simulink library "BF_MASTER"  (Simulink 8.6)
settings: Solver=ode45  StartTime=0.0  StopTime=10.0  RelTol=1e-3
libraries: cdsEpicsOut x60, cdsFilt x51, cdsFiltCtrl x28, cdsTP x28, cdsEpicsIn x14, cdsMuxMatrix x6, VIS_LIB x5, cdsEpicsBinIn x3, cdsOsc x2, cdsFunctionCall x2, SIXOSEM_F_STAGE_MASTER x2, CRYP_IM_MASTER x1
(part 5 of 9)

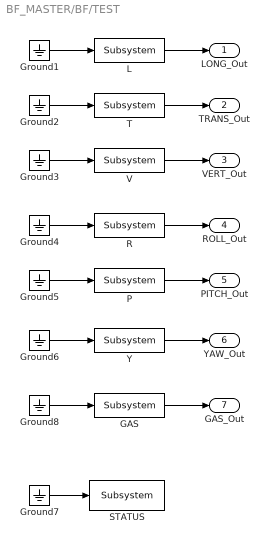
== system BF_MASTER/BF/TEST ==
  GAS : cdsFilt/Subsystem  Tag=cdsFilt  Description=|
      | Purpose:                                                                                                                                                                                                                                  
      | Standard CDS IIR filter module.                                                                                                                                                                                                           
      |                                                                                                                                                                                                                                           
      | Operation:                                                                                                                                                                                                                                
      | Consists of 10 second order section IIR filters, plus a ramped gain stage. In FE code, also provides pre-defined test points and excitation channel inputs. The filter coefficients are defined in the LIGO system using the 'foton' tool.
      |                                                                                                                                                                                                                                           
      | Usage:                                                                                                                                                                                                                                    
      | Name the part with the desired filter module name.
      settings: AttributesFormatString=%<Tag>
  Ground{1..8} (8 alike) : Ground
  L : cdsFilt/Subsystem  Tag=cdsFilt  Description=|
      | Purpose:                                                                                                                                                                                                                                  
      | Standard CDS IIR filter module.                                                                                                                                                                                                           
      |                                                                                                                                                                                                                                           
      | Operation:                                                                                                                                                                                                                                
      | Consists of 10 second order section IIR filters, plus a ramped gain stage. In FE code, also provides pre-defined test points and excitation channel inputs. The filter coefficients are defined in the LIGO system using the 'foton' tool.
      |                                                                                                                                                                                                                                           
      | Usage:                                                                                                                                                                                                                                    
      | Name the part with the desired filter module name.
      settings: AttributesFormatString=%<Tag>
  P : cdsFilt/Subsystem  Tag=cdsFilt  Description=|
      | Purpose:                                                                                                                                                                                                                                  
      | Standard CDS IIR filter module.                                                                                                                                                                                                           
      |                                                                                                                                                                                                                                           
      | Operation:                                                                                                                                                                                                                                
      | Consists of 10 second order section IIR filters, plus a ramped gain stage. In FE code, also provides pre-defined test points and excitation channel inputs. The filter coefficients are defined in the LIGO system using the 'foton' tool.
      |                                                                                                                                                                                                                                           
      | Usage:                                                                                                                                                                                                                                    
      | Name the part with the desired filter module name.
      settings: AttributesFormatString=%<Tag>
  R : cdsFilt/Subsystem  Tag=cdsFilt  Description=|
      | Purpose:                                                                                                                                                                                                                                  
      | Standard CDS IIR filter module.                                                                                                                                                                                                           
      |                                                                                                                                                                                                                                           
      | Operation:                                                                                                                                                                                                                                
      | Consists of 10 second order section IIR filters, plus a ramped gain stage. In FE code, also provides pre-defined test points and excitation channel inputs. The filter coefficients are defined in the LIGO system using the 'foton' tool.
      |                                                                                                                                                                                                                                           
      | Usage:                                                                                                                                                                                                                                    
      | Name the part with the desired filter module name.
      settings: AttributesFormatString=%<Tag>
  STATUS : cdsEpicsBinIn/Subsystem  Tag=cdsEpicsBinIn  Description=|
      | Purpose:                                                                            
      | Create an EPICS binary (0 or 1) input channel to the FE realtime controls.          
      |                                                                                     
      | Operation:                                                                          
      | Outputs value from an EPICS ai record. Value is binary input (bi Epics record type).
      |                                                                                     
      | Usage:                                                                              
      | Name the part with the desired EPICS channel name.
      settings: AttributesFormatString=%<Tag>
  T : cdsFilt/Subsystem  Tag=cdsFilt  Description=|
      | Purpose:                                                                                                                                                                                                                                  
      | Standard CDS IIR filter module.                                                                                                                                                                                                           
      |                                                                                                                                                                                                                                           
      | Operation:                                                                                                                                                                                                                                
      | Consists of 10 second order section IIR filters, plus a ramped gain stage. In FE code, also provides pre-defined test points and excitation channel inputs. The filter coefficients are defined in the LIGO system using the 'foton' tool.
      |                                                                                                                                                                                                                                           
      | Usage:                                                                                                                                                                                                                                    
      | Name the part with the desired filter module name.
      settings: AttributesFormatString=%<Tag>
  V : cdsFilt/Subsystem  Tag=cdsFilt  Description=|
      | Purpose:                                                                                                                                                                                                                                  
      | Standard CDS IIR filter module.                                                                                                                                                                                                           
      |                                                                                                                                                                                                                                           
      | Operation:                                                                                                                                                                                                                                
      | Consists of 10 second order section IIR filters, plus a ramped gain stage. In FE code, also provides pre-defined test points and excitation channel inputs. The filter coefficients are defined in the LIGO system using the 'foton' tool.
      |                                                                                                                                                                                                                                           
      | Usage:                                                                                                                                                                                                                                    
      | Name the part with the desired filter module name.
      settings: AttributesFormatString=%<Tag>
  Y : cdsFilt/Subsystem  Tag=cdsFilt  Description=|
      | Purpose:                                                                                                                                                                                                                                  
      | Standard CDS IIR filter module.                                                                                                                                                                                                           
      |                                                                                                                                                                                                                                           
      | Operation:                                                                                                                                                                                                                                
      | Consists of 10 second order section IIR filters, plus a ramped gain stage. In FE code, also provides pre-defined test points and excitation channel inputs. The filter coefficients are defined in the LIGO system using the 'foton' tool.
      |                                                                                                                                                                                                                                           
      | Usage:                                                                                                                                                                                                                                    
      | Name the part with the desired filter module name.
      settings: AttributesFormatString=%<Tag>
  LONG_Out : Outport
  TRANS_Out : Outport  Port=2
  VERT_Out : Outport  Port=3
  ROLL_Out : Outport  Port=4
  PITCH_Out : Outport  Port=5
  YAW_Out : Outport  Port=6
  GAS_Out : Outport  Port=7
  wires:
  L/1 -> LONG_Out/1
  T/1 -> TRANS_Out/1
  V/1 -> VERT_Out/1
  Y/1 -> YAW_Out/1
  P/1 -> PITCH_Out/1
  R/1 -> ROLL_Out/1
  Ground1/1 -> L/1
  Ground2/1 -> T/1
  Ground3/1 -> V/1
  Ground6/1 -> Y/1
  Ground5/1 -> P/1
  Ground4/1 -> R/1
  Ground7/1 -> STATUS/1
  GAS/1 -> GAS_Out/1
  Ground8/1 -> GAS/1

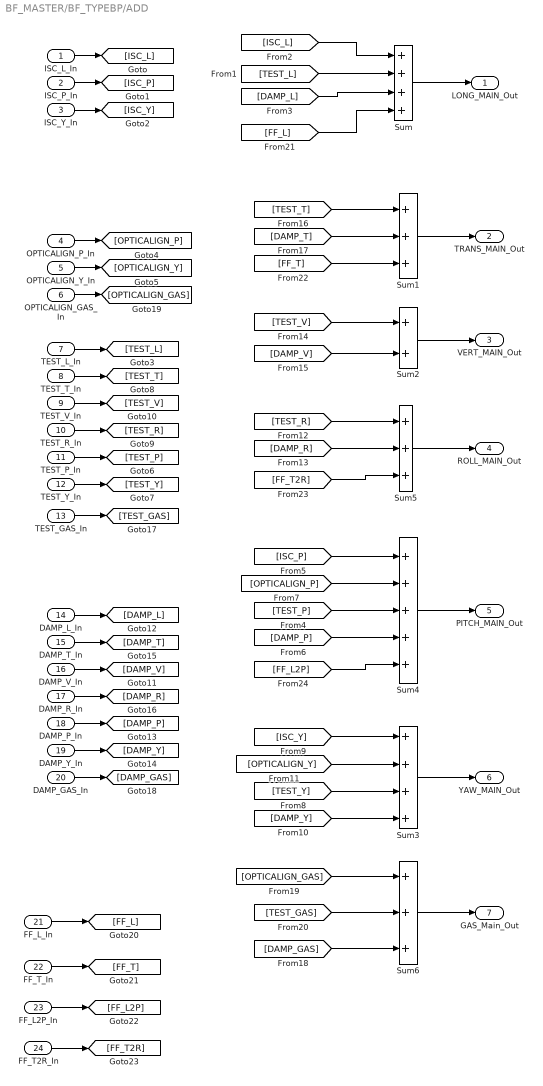
== system BF_MASTER/BF_TYPEBP/ADD ==
  ISC_L_In : Inport
  ISC_P_In : Inport  Port=2
  ISC_Y_In : Inport  Port=3
  OPTICALIGN_P_In : Inport  Port=4
  OPTICALIGN_Y_In : Inport  Port=5
  OPTICALIGN_GAS_In : Inport  Port=6
  TEST_L_In : Inport  Port=7
  TEST_T_In : Inport  Port=8
  TEST_V_In : Inport  Port=9
  TEST_R_In : Inport  Port=10
  TEST_P_In : Inport  Port=11
  TEST_Y_In : Inport  Port=12
  TEST_GAS_In : Inport  Port=13
  DAMP_L_In : Inport  Port=14
  DAMP_T_In : Inport  Port=15
  DAMP_V_In : Inport  Port=16
  DAMP_R_In : Inport  Port=17
  DAMP_P_In : Inport  Port=18
  DAMP_Y_In : Inport  Port=19
  DAMP_GAS_In : Inport  Port=20
  FF_L_In : Inport  Port=21
  FF_T_In : Inport  Port=22
  FF_L2P_In : Inport  Port=23
  FF_T2R_In : Inport  Port=24
  Sum : Sum  Inputs=++++
  Sum1 : Sum  Inputs=+++
  Sum2 : Sum
  Sum3 : Sum  Inputs=++++
  Sum4 : Sum  Inputs=+++++
  Sum5 : Sum  Inputs=+++
  Sum6 : Sum  Inputs=+++
  LONG_MAIN_Out : Outport
  TRANS_MAIN_Out : Outport  Port=2
  VERT_MAIN_Out : Outport  Port=3
  ROLL_MAIN_Out : Outport  Port=4
  PITCH_MAIN_Out : Outport  Port=5
  YAW_MAIN_Out : Outport  Port=6
  GAS_Main_Out : Outport  Port=7
  wires:
  [DAMP_V] -> Sum2/2
  [TEST_V] -> Sum2/1
  [DAMP_T] -> Sum1/2
  [TEST_T] -> Sum1/1
  [DAMP_R] -> Sum5/2
  [TEST_R] -> Sum5/1
  [DAMP_Y] -> Sum3/4
  [TEST_Y] -> Sum3/3
  [OPTICALIGN_Y] -> Sum3/2
  [ISC_Y] -> Sum3/1
  [DAMP_P] -> Sum4/4
  [TEST_P] -> Sum4/3
  [OPTICALIGN_P] -> Sum4/2
  [ISC_P] -> Sum4/1
  ISC_Y_In/1 -> [ISC_Y]
  ISC_P_In/1 -> [ISC_P]
  ISC_L_In/1 -> [ISC_L]
  OPTICALIGN_Y_In/1 -> [OPTICALIGN_Y]
  OPTICALIGN_P_In/1 -> [OPTICALIGN_P]
  Sum1/1 -> TRANS_MAIN_Out/1
  Sum2/1 -> VERT_MAIN_Out/1
  Sum5/1 -> ROLL_MAIN_Out/1
  [DAMP_L] -> Sum/3
  [TEST_L] -> Sum/2
  [ISC_L] -> Sum/1
  Sum/1 -> LONG_MAIN_Out/1
  Sum3/1 -> YAW_MAIN_Out/1
  Sum4/1 -> PITCH_MAIN_Out/1
  Sum6/1 -> GAS_Main_Out/1
  OPTICALIGN_GAS_In/1 -> [OPTICALIGN_GAS]
  TEST_L_In/1 -> [TEST_L]
  TEST_T_In/1 -> [TEST_T]
  TEST_V_In/1 -> [TEST_V]
  TEST_R_In/1 -> [TEST_R]
  TEST_P_In/1 -> [TEST_P]
  TEST_Y_In/1 -> [TEST_Y]
  TEST_GAS_In/1 -> [TEST_GAS]
  DAMP_L_In/1 -> [DAMP_L]
  DAMP_T_In/1 -> [DAMP_T]
  DAMP_V_In/1 -> [DAMP_V]
  DAMP_R_In/1 -> [DAMP_R]
  DAMP_P_In/1 -> [DAMP_P]
  DAMP_Y_In/1 -> [DAMP_Y]
  DAMP_GAS_In/1 -> [DAMP_GAS]
  [OPTICALIGN_GAS] -> Sum6/1
  [TEST_GAS] -> Sum6/2
  [DAMP_GAS] -> Sum6/3
  FF_L_In/1 -> [FF_L]
  FF_T_In/1 -> [FF_T]
  [FF_L] -> Sum/4
  [FF_T] -> Sum1/3
  FF_L2P_In/1 -> [FF_L2P]
  [FF_T2R] -> Sum5/3
  [FF_L2P] -> Sum4/5
  FF_T2R_In/1 -> [FF_T2R]
